simulink model "ArtificialDampingforThetaControl"  (R2018b)
settings: Solver=VariableStepAuto  StartTime=0.0  StopTime=100  RelTol=1e-3
settings Model: Creator=cdjsd  LastModifiedBy=cdjsd

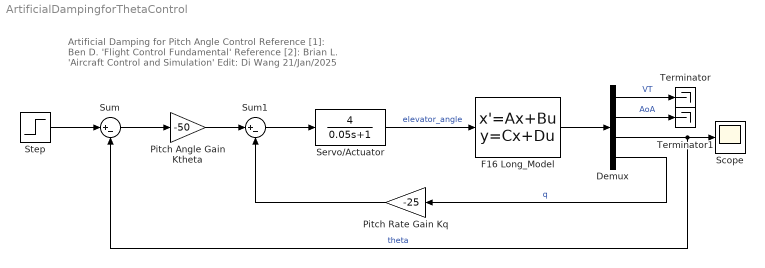
== system ArtificialDampingforThetaControl ==
  note: Artificial Damping for Pitch Angle Control
      | Reference [1]: Ben D. 'Flight Control Fundamental'
      | Reference [2]: Brian L. 'Aircraft Control and Simulation'
      | Edit: Di Wang 21/Jan/2025
  Demux : Demux
  F16 Long_Model : StateSpace  A=|  B=|  C=eye(4)  D=zeros(4,1)  InitialCondition=0
      A=|
      | [-1.9311e-2 8.8157 -3.217e1 -5.7499e-1;
      |      -2.5389e-4 -1.0189 0 9.0506e-1;
      |      0 0 0 1;
      |      2.9465e-12 8.2225e-1 0 -1.0744]
      B=|
      | [1.737e-1;
      |      -2.1499e-3;
      |      0;
      |      -1.7555e-1]
  Pitch Angle Gain Ktheta : Gain  Gain=-50
  Pitch Rate Gain Kq : Gain  Gain=-25
  Scope : Scope
  Servo/Actuator : TransferFcn  Numerator=4  Denominator=[0.05 1]
  Step : Step  SampleTime=0
  Sum : Sum  Inputs=|+-
  Sum1 : Sum  Inputs=|+-
  Terminator : Terminator
  Terminator1 : Terminator
  wires:
  Step/1 -> Sum/1
  Sum/1 -> Pitch Angle Gain Ktheta/1
  Pitch Angle Gain Ktheta/1 -> Sum1/1
  Servo/Actuator/1 -> F16 Long_Model/1  "elevator_angle"
  F16 Long_Model/1 -> Demux/1
  Sum1/1 -> Servo/Actuator/1
  Pitch Rate Gain Kq/1 -> Sum1/2
  Demux/3 -> Sum/2, Scope/1  "theta"
  Demux/4 -> Pitch Rate Gain Kq/1  "q"
  Demux/1 -> Terminator/1  "VT"
  Demux/2 -> Terminator1/1  "AoA"
